simulink model "iir"  (Simulink 7.2)
settings: Solver=ode45  StartTime=0.0  StopTime=10.0  RelTol=1e-3
settings Model: Creator=dsgib  LastModifiedBy=dsgib

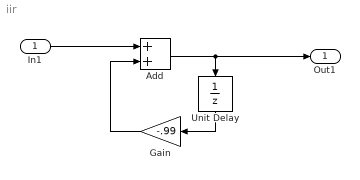
== system iir ==
  In1 : Inport  OutDataType=sfix(16)  OutScaling=2^0
  Add : Sum  OutDataType=sfix(16)  OutScaling=2^-10
  Gain : Gain  Orientation=left  Gain=-.99  ParameterDataType=sfix(16)  ParameterScaling=2^0  OutDataType=sfix(16)  OutScaling=2^0
  Unit Delay : UnitDelay  Orientation=down
  Out1 : Outport  OutDataType=sfix(16)  OutScaling=2^0
  wires:
  In1/1 -> Add/1
  Add/1 -> Out1/1, Unit Delay/1
  Unit Delay/1 -> Gain/1
  Gain/1 -> Add/2
